simulink model "OpenLoopSystemSimulation.png"  (R2024b)
settings: Solver=VariableStepAuto  StartTime=0.0  StopTime=20  RelTol=1e-3
undefined symbols (not defined in the file): btm, Jm, Ktm, Kv, Lm, R
settings Model: Creator=mwali  LastModifiedBy=user
settings RTWCC: GPUComputeCapability=3.5

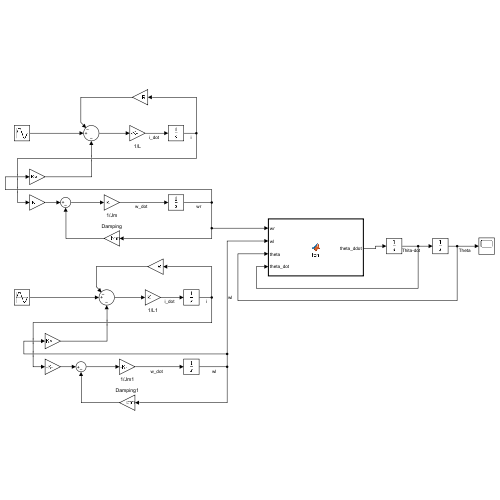
[thumbnail: Simulink's stored preview of the top-level diagram]
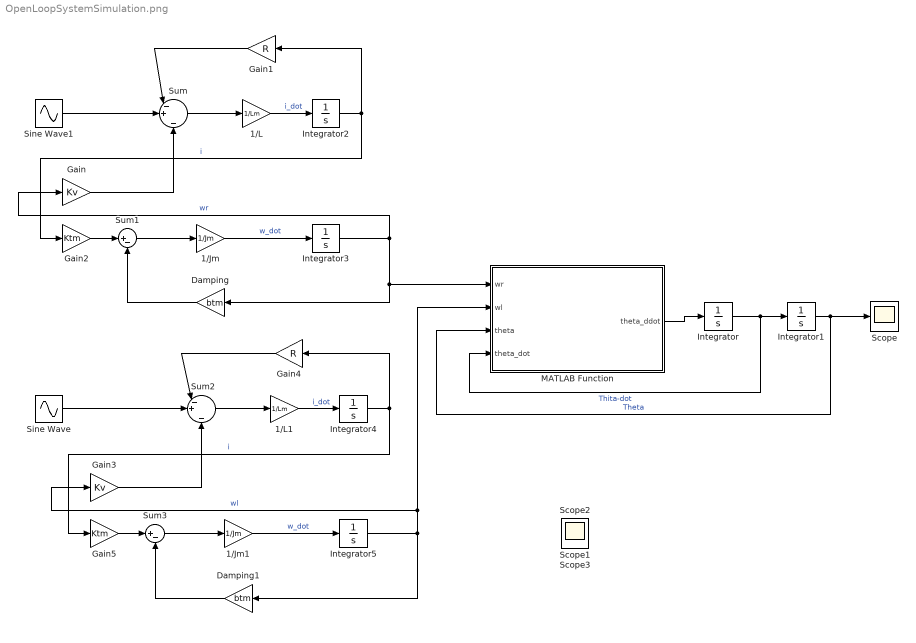
== system OpenLoopSystemSimulation.png ==
  1/Jm : Gain  Gain=1/Jm
  1/Jm1 : Gain  Gain=1/Jm
  1/L : Gain  Gain=1/Lm
  1/L1 : Gain  Gain=1/Lm
  Damping : Gain  Gain=btm
  Damping1 : Gain  Gain=btm
  Gain : Gain  Gain=Kv
  Gain1 : Gain  Gain=R
  Gain2 : Gain  Gain=Ktm
  Gain3 : Gain  Gain=Kv
  Gain4 : Gain  Gain=R
  Gain5 : Gain  Gain=Ktm
  Integrator{,1..5} (6 alike) : Integrator
  MATLAB Function : MATLAB Function  TreatAsAtomicUnit=on
  Scope{,1..3} (4 alike) : Scope
  Sine Wave : Sin  SampleTime=0
  Sine Wave1 : Sin  Amplitude=5  SampleTime=0
  Sum : Sum  Inputs=|-+|-
  Sum1 : Sum  Inputs=|+-
  Sum2 : Sum  Inputs=|-+|-
  Sum3 : Sum  Inputs=|+-
  wires:
  MATLAB Function/1(theta_ddot) -> Integrator/1
  Integrator/1 -> MATLAB Function/4(theta_dot), Integrator1/1  "Thita-dot"
  Integrator1/1 -> MATLAB Function/3(theta), Scope/1  "Theta"
  Sine Wave1/1 -> Sum/2
  1/L/1 -> Integrator2/1  "i_dot"
  Integrator2/1 -> Gain2/1, Gain1/1  "i"
  Sum/1 -> 1/L/1
  Gain/1 -> Sum/3
  Gain2/1 -> Sum1/1
  Sum1/1 -> 1/Jm/1
  1/Jm/1 -> Integrator3/1  "w_dot"
  Integrator3/1 -> Gain/1, MATLAB Function/1(wr), Damping/1  "wr"
  Sum3/1 -> 1/Jm1/1
  Integrator4/1 -> Gain5/1, Gain4/1  "i"
  1/L1/1 -> Integrator4/1  "i_dot"
  Gain5/1 -> Sum3/1
  Gain4/1 -> Sum2/1
  Integrator5/1 -> Gain3/1, MATLAB Function/2(wl), Damping1/1  "wl"
  Gain3/1 -> Sum2/3
  Sine Wave/1 -> Sum2/2
  Sum2/1 -> 1/L1/1
  1/Jm1/1 -> Integrator5/1  "w_dot"
  Gain1/1 -> Sum/1
  Damping/1 -> Sum1/2
  Damping1/1 -> Sum3/2

== matlab function OpenLoopSystemSimulation.png/MATLAB Function ==
  data: wr input; theta_ddot output; wl input; theta input; theta_dot input
function theta_ddot  = fcn(wr,wl,theta,theta_dot)
   
  L= 600e-3;
  Kt = 100e-6;
  Wo  = 2.0;        
  Lb = 300e-3;
  mb = 75e-3;
  g   = 9.81;
  J = 58.23e-3;
  bt = 10e-3;


    theta_ddot = ((2*L*Kt*Wo * (wr - wl)) - (bt * theta_dot) - ((Lb/2) * mb * g *  theta)) / J;
end
